simulink model "porovnani_modelu"  (R2023a)
settings: Solver=ode4  StartTime=0.0  StopTime=15  FixedStep=1e-3  RelTol=1e-3
values from neighbouring files (symbols this model uses):
  d = 0.1    [parametry_Lagrange.m]    (also in parametry_a_vizualizace.m)
  g = 9.81    [parametry_Lagrange.m]    (also in parametry_a_vizualizace.m)
  Ikv = 0.00025    [parametry_Lagrange.m]    (also in parametry_a_vizualizace.m)
  Ip = m*d^2    (= 0.0001)    [parametry_Lagrange.m]    (also in parametry_a_vizualizace.m)
  k = 0    [parametry_Lagrange.m]    (also in parametry_a_vizualizace.m = 0.1)
  kp = 0    [parametry_Lagrange.m]    (also in parametry_a_vizualizace.m = 0.01)
  L = 0.086    [parametry_Lagrange.m]    (also in parametry_a_vizualizace.m)
  M = 0.5    [parametry_Lagrange.m]    (also in parametry_a_vizualizace.m)
  m = 0.01    [parametry_Lagrange.m]    (also in parametry_a_vizualizace.m)
libraries: simulink_extras x2
settings Model: PacingRate=5  Creator=Admin  LastModifiedBy=Admin

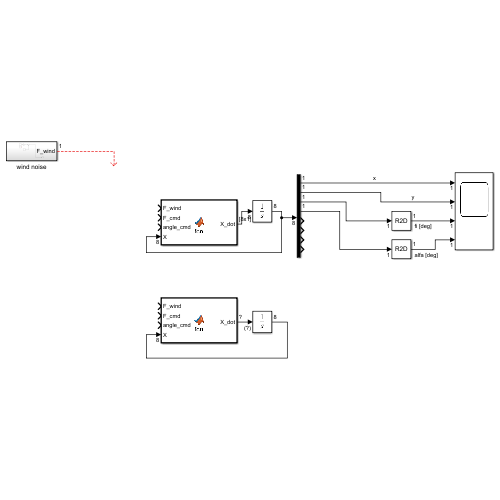
[thumbnail: Simulink's stored preview of the top-level diagram]
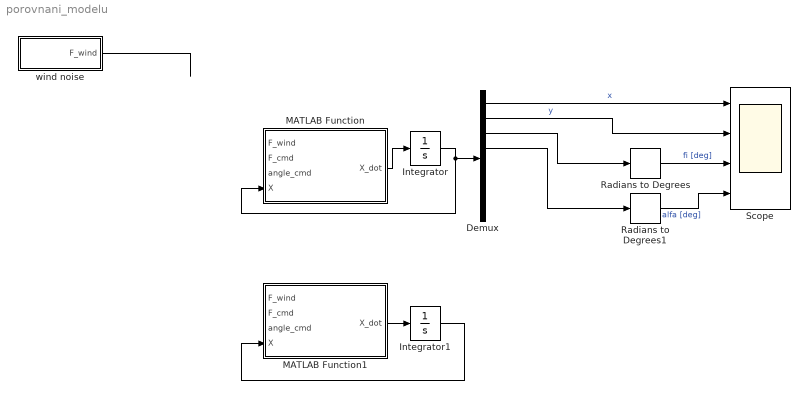
== system porovnani_modelu ==
  Demux : Demux  Outputs=8
  Integrator : Integrator  InitialCondition=[0;0;0;0;0;0;0;0]  UpperSaturationLimit=[inf; inf; inf; pi; inf; inf; inf; inf]  LowerSaturationLimit=[-inf; -inf; -inf; -pi; -inf; -inf; -inf; -inf]  IgnoreLimit=on
  Integrator1 : Integrator  InitialCondition=[0;0;0;0;0;0;0;0]  UpperSaturationLimit=[inf; inf; inf; pi; inf; inf; inf; inf]  LowerSaturationLimit=[-inf; -inf; -inf; -pi; -inf; -inf; -inf; -inf]  IgnoreLimit=on
  MATLAB Function : MATLAB Function  TreatAsAtomicUnit=on
  MATLAB Function1 : MATLAB Function  TreatAsAtomicUnit=on
  Radians to Degrees : simulink_extras/Transformations/Radians to Degrees
  Radians to Degrees1 : simulink_extras/Transformations/Radians to Degrees
  Scope : Scope  NumInputPorts=4
  wind noise : Subsystem
  wires:
  MATLAB Function/1(X_dot) -> Integrator/1
  Integrator/1 -> MATLAB Function/4(X), Demux/1
  Demux/3 -> Radians to Degrees/1
  Demux/2 -> Scope/2  "y"
  Demux/1 -> Scope/1  "x"
  Radians to Degrees/1 -> Scope/3  "fi [deg]"
  Demux/4 -> Radians to Degrees1/1
  Radians to Degrees1/1 -> Scope/4  "alfa [deg]"
  wind noise/1(F_wind) -> ?
  MATLAB Function1/1(X_dot) -> Integrator1/1
  Integrator1/1 -> MATLAB Function1/4(X)

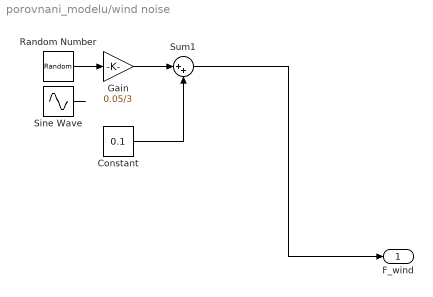
== system porovnani_modelu/wind noise ==
  Constant : Constant  Value=0.1
  Gain : Gain  Gain=0.05/3
  Random Number : RandomNumber  SampleTime=0.1
  Sine Wave : Sin  Amplitude=0.1  Frequency=0.5  SampleTime=0
  Sum1 : Sum  Inputs=|++
  F_wind : Outport
  wires:
  Sum1/1 -> F_wind/1
  Gain/1 -> Sum1/1
  Sine Wave/1 -> ?
  Random Number/1 -> Gain/1
  Constant/1 -> Sum1/2

== matlab function porovnani_modelu/MATLAB Function1 ==
  data: F_wind input; F_cmd input; angle_cmd input; X_dot output; X input; g parameter; L parameter; d parameter; M parameter; m parameter; Ikv parameter; Ip parameter; k parameter; kp parameter
function X_dot = fcn(F_wind, F_cmd, angle_cmd, X, g, L, d, M, m, Ikv, Ip, k, kp)
% [x1, x2, x3, x4, x5, x6, x7, x8] = [x, y, fi, alfa, x_dot, y_dot, fi_dot, alfa_dot]
x1 = X(1);
x2 = X(2);
x3 = X(3);
x4 = X(4);
x5 = X(5);
x6 = X(6);
x7 = X(7);
x8 = X(8);

F1 = F_cmd + angle_cmd; % Celková tažná síla na 1. motoru
F2 = F_cmd - angle_cmd; % Celková tažná síla na 2. motoru
% F1 a F2 lze také vyjádřit přes úhlové rychlosti motorů, např.
% w1 = F_cmd + angle_cmd
% w2 = F_cmd - angle_cmd
% F1 = koef * w1^2; F2 = koef * w2^2


x1_dot = x5;
x2_dot = x6;
x3_dot = x7;
x4_dot = x8;

x5_dot = -(sin(x3)*(F1 + F2) - F_wind + k*x5 + kp*(x5 + d*x8*cos(x4)) + m*(d*x8_dot*cos(x4) - d*x8^2*sin(x4)))/(M + m);
x6_dot = -(M*g - cos(x3)*(F1 + F2) + g*m + k*x6 + m*(d*cos(x4)*x8^2 + d*x8_dot*sin(x4)) + kp*(x6 + d*x8*sin(x4)))/(M + m);
x7_dot = (F1-F2)*L/Ikv;

x8_dot = -(d^2*kp*x8*cos(x4)^2 + d^2*kp*x8*sin(x4)^2 + d*kp*x5*cos(x4) + d*g*m*sin(x4) + d*m*x5_dot*cos(x4) + d*kp*x6*sin(x4) + d*m*x6_dot*sin(x4))/(m*d^2*cos(x4)^2 + m*d^2*sin(x4)^2 + m*d^2);

X_dot = [x1_dot, x2_dot, x3_dot, x4_dot, x5_dot, x6_dot, x7_dot, x8_dot]';

== matlab function porovnani_modelu/MATLAB Function ==
  data: F_wind input; F_cmd input; angle_cmd input; X_dot output; X input; g parameter; L parameter; d parameter; M parameter; m parameter; Ikv parameter; Ip parameter; k parameter; kp parameter
function X_dot = fcn(F_wind, F_cmd, angle_cmd, X, g, L, d, M, m, Ikv, Ip, k, kp)
% [x1, x2, x3, x4, x5, x6, x7, x8] = [x, y, fi, alfa, x_dot, y_dot, fi_dot, alfa_dot]
x1 = X(1);
x2 = X(2);
x3 = X(3);
x4 = X(4);
x5 = X(5);
x6 = X(6);
x7 = X(7);
x8 = X(8);

F1 = F_cmd + angle_cmd; % Celková tažná síla na 1. motoru
F2 = F_cmd - angle_cmd; % Celková tažná síla na 2. motoru
% F1 a F2 lze také vyjádřit přes úhlové rychlosti motorů, např.
% w1 = F_cmd + angle_cmd
% w2 = F_cmd - angle_cmd
% F1 = koef * w1^2; F2 = koef * w2^2


x1_dot = x5;
x2_dot = x6;
x3_dot = x7;
x4_dot = x8;

%x5_dot = -(sin(x3)*(F1 + F2) - F_wind + k*x5 + kp*(x5 + d*x8*cos(x4)) - m*(d*x8^2*sin(x4) - (d*g*m*cos(x4)*sin(x4))/Ip))/(M + m);
x5_dot = -(sin(x3)*(F1 + F2) - F_wind - m*(d*x8^2*sin(x4) - g*cos(x4)*sin(x4)) + k*x5 + kp*(x5 + d*x8*cos(x4)))/(M + m);
%x6_dot = -(M*g - cos(x3)*(F1 + F2) + m*(d*x8^2*cos(x4) + (d*g*m*sin(x4)^2)/Ip) + g*m + k*x6 + kp*(x6 + d*x8*sin(x4)))/(M + m);
x6_dot = -(M*g - cos(x3)*(F1 + F2) + g*m + k*x6 + m*(d*cos(x4)*x8^2 + g*sin(x4)^2) + kp*(x6 + d*x8*sin(x4)))/(M + m);
x7_dot = (F1-F2)*L/Ikv;

%x8_dot = -(kp*x5*cos(x4) + g*m*sin(x4) + kp*x6*sin(x4) + d*kp*x8 - (m*cos(x4)*(sin(x3)*(F1 + F2) - F_wind + k*x5 + kp*(x5 + d*x8*cos(x4)) - m*(d*x8^2*sin(x4) - (d*g*m*cos(x4)*sin(x4))/Ip)))/(M + m) - (m*sin(x4)*(M*g - cos(x3)*(F1 + F2) + m*(d*x8^2*cos(x4) + (d*g*m*sin(x4)^2)/Ip) + g*m + k*x6 + kp*(x6 + d*x8*sin(x4))))/(M + m))/(d*m);
x8_dot = -(kp*x5*cos(x4) + g*m*sin(x4) + kp*x6*sin(x4) + d*kp*x8 - (m*cos(x4)*(sin(x3)*(F1 + F2) - F_wind - m*(d*x8^2*sin(x4) - g*cos(x4)*sin(x4)) + k*x5 + kp*(x5 + d*x8*cos(x4))))/(M + m) - (m*sin(x4)*(M*g - cos(x3)*(F1 + F2) + g*m + k*x6 + m*(d*cos(x4)*x8^2 + g*sin(x4)^2) + kp*(x6 + d*x8*sin(x4))))/(M + m))/(d*m);

X_dot = [x1_dot, x2_dot, x3_dot, x4_dot, x5_dot, x6_dot, x7_dot, x8_dot]';
